simulink model "Assignment_2_1_simulink"  (R2025a)
settings: Solver=FixedStepDiscrete  StartTime=0.0  StopTime=inf  FixedStep=0.1  RelTol=1e-3  EnableMultiTasking=on
model workspace (MAT data in the model file):
  Logfile_Data_Object : ros2bag (value not decoded)
  Logfile_Path = '/home/diego/Desktop/Assignments/GitHub/ASSIGNMENT_2/tb3_subset/metadata.yaml'
  Logfile_Playback_Duration = nan
  Logfile_Playback_Offset = nan
values from neighbouring files (symbols this model uses):
  Kv = 0.8    [Assignment_2.m]
  Kw = 2    [Assignment_2.m]
  Quaternion_Matrix = [waypoints(:, 1:2) Quaternion_Matrix]    [Assignment_2.m]
  tol = 0.05    [Assignment_2.m]
undefined symbols (not defined in the file or in its folder): twist
libraries: ros2lib x5
settings Model: Creator=arrigon88_msi_u24  LastModifiedBy=diego
settings OptimizationCC: DefaultParameterBehavior=Inlined  EnhancedBackFolding=on  PassReuseOutputArgsAs=Individual arguments  ZeroExternalMemoryAtStartup=off  ZeroInternalMemoryAtStartup=off  MaxStackSize=64  OptimizeBlockOrder=speed  DifferentSizesBufferReuse=on  OptimizationCustomize=off  EfficientTunableParamExpr=on
settings DebuggingCC: ParameterTunabilityLossMsg=error
settings HardwareCC: ProdBitPerLong=64.0  ProdHWDeviceType=Intel->x86-64 (Linux 64)
settings SFSimCC: MATLABDynamicMemAlloc=off
settings RTWCC: SystemTargetFile=ert.tlc  HardwareBoard=Robot Operating System 2 (ROS 2)  TLCOptions="-aInlineSetEventsForThisBaseRateFcn=TLC_FALSE -aSuppressMultiTaskScheduler=TLC_FALSE  -aRateBasedStepFcn=0"  TemplateMakefile=ert_default_tmf  Toolchain=Colcon Tools  TargetLang=C++  Description=Embedded Coder
settings CodeAppCC: ForceParamTrailComments=on  IgnoreCustomStorageClasses=off  OperatorAnnotations=on  SimulinkDataObjDesc=on  SFDataObjDesc=on  InsertBlockDesc=on
settings ERTTargetCC: ExtModeTransport=2.0  ExtModeAutomaticAllocSize=off  RootIOFormat=Structure reference  CodeInterfacePackaging=C++ class

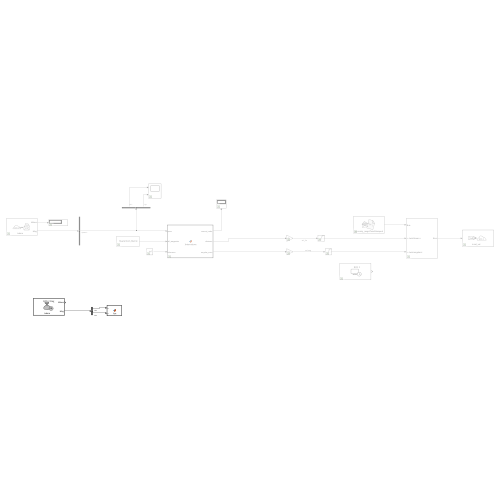
[thumbnail: Simulink's stored preview of the top-level diagram]
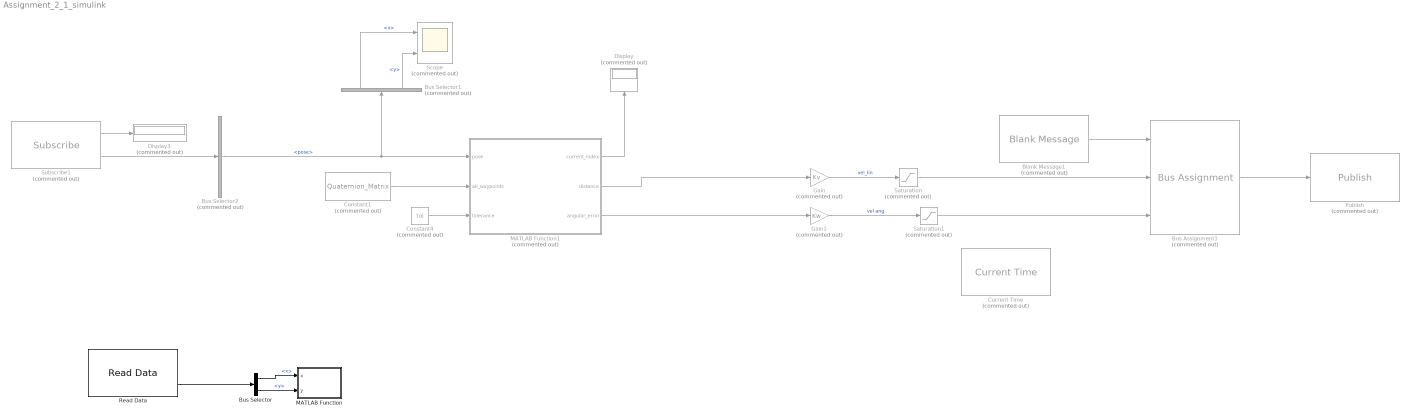
== system Assignment_2_1_simulink ==
  Blank Message1 : ros2lib/Blank Message  Commented=on  messageClass=Message  entityType=geometry_msgs/TwistStamped  messageType=geometry_msgs/TwistStamped  SampleTime=inf
  Bus Assignment1 : BusAssignment  Commented=on  AssignedSignals=twist.linear.x,twist.angular.z
  Bus Selector : BusSelector  OutputSignals=pose.pose.position.x,pose.pose.position.y
  Bus Selector1 : BusSelector  Commented=on  OutputSignals=pose.position.x,pose.position.y
  Bus Selector2 : BusSelector  Commented=on  OutputSignals=pose
  Constant1 : Constant  Commented=on  Value=Quaternion_Matrix
  Constant4 : Constant  Commented=on  Value=tol
  Current Time : ros2lib/Current Time  Commented=on  OutputFormat=double  SampleTime=-1  ModelName=Assignment_2_simulink
  Display : Display  Commented=on
  Display3 : Display  Commented=on
  Gain : Gain  Commented=on  Gain=Kv
  Gain1 : Gain  Commented=on  Gain=Kw
  MATLAB Function : MATLAB Function  TreatAsAtomicUnit=on
  MATLAB Function1 : MATLAB Function  Commented=on  TreatAsAtomicUnit=on
  Publish : ros2lib/Publish  Commented=on  topicSource=Select from ROS network  topic=/cmd_vel  messageType=geometry_msgs/TwistStamped  QOSHistory=Keep last  QOSDepth=10  QOSReliability=Reliable  QOSDurability=Volatile  QOSDeadline=Inf  QOSLifespan=Inf  QOSLiveliness=Automatic  QOSLeaseDuration=Inf  QOSAvoidROSNamespaceConventions=off
  Read Data : ros2lib/Read Data  topic=/odom  sampleTime=-1  logfileType=rosbag2  modelName=Assignment_2_1_simulink  msgType=nav_msgs/Odometry
  Saturation : Saturate  Commented=on  UpperLimit=0.2  LowerLimit=0
  Saturation1 : Saturate  Commented=on  UpperLimit=0.4  LowerLimit=0
  Scope : Scope  Commented=on  NumInputPorts=2
      settings: ActiveDisplayYMinimum=-7.8774180960192659  ActiveDisplayYMaximum=6.4713068809857548
  Subscribe1 : ros2lib/Subscribe  Commented=on  topicSource=Select from ROS network  topic=/odom  messageType=nav_msgs/Odometry  sampleTime=-1  QOSHistory=Keep last  QOSDepth=10  QOSReliability=Reliable  QOSDurability=Volatile  QOSDeadline=Inf  QOSLifespan=Inf  QOSLiveliness=Automatic  QOSLeaseDuration=Inf  QOSAvoidROSNamespaceConventions=off
  wires:
  MATLAB Function1/1(current_index) -> Display/1
  Subscribe1/2 -> Bus Selector2/1
  Subscribe1/1 -> Display3/1
  Constant4/1 -> MATLAB Function1/3(tolerance)
  MATLAB Function1/2(distance) -> Gain/1
  Gain/1 -> Saturation/1  "vel_lin"
  MATLAB Function1/3(angular_error) -> Gain1/1
  Gain1/1 -> Saturation1/1  "vel ang"
  Saturation/1 -> Bus Assignment1/2
  Blank Message1/1 -> Bus Assignment1/1
  Bus Assignment1/1 -> Publish/1
  Saturation1/1 -> Bus Assignment1/3
  Bus Selector2/1 -> Bus Selector1/1, MATLAB Function1/1(pose)  "<pose>"
  Bus Selector1/2 -> Scope/2  "<y>"
  Bus Selector1/1 -> Scope/1  "<x>"
  Constant1/1 -> MATLAB Function1/2(all_waypoints)
  Read Data/2 -> Bus Selector/1
  Bus Selector/1 -> MATLAB Function/1(x)  "<x>"
  Bus Selector/2 -> MATLAB Function/2(y)  "<y>"

== matlab function Assignment_2_1_simulink/MATLAB Function1 ==
  data: pose input; current_index output; all_waypoints input; tolerance input; distance output; angular_error output
function [current_index, distance, angular_error] = Interruttore(pose, all_waypoints, tolerance)
    
   % -----------------------------------------------------------------
    
    % Dichiara 'index' come persistente (mantiene il valore tra le chiamate)
    persistent index;
    
    % Inizializza 'index' solo alla prima chiamata (quando e' vuoto)
    if isempty(index)
        index = 1; % Inizia dal primo waypoint
    end

    % Ottieni il numero totale di waypoint per sicurezza
    num_waypoints = size(all_waypoints, 1);

    % Assicurati che l'indice non superi il massimo
    % (se siamo arrivati all'ultimo, rimaniamo li)
    if index > num_waypoints
        index = num_waypoints;
    end
    
    % -----------------------------------------------------------------
    % 2. ESECUZIONE LOGICA
    % -----------------------------------------------------------------
    
    % Estrai il target CORRENTE usando l'indice interno
    target = all_waypoints(index, :);
    
    % Assegna l'output: 'current_index' e' l'indice che stiamo processando
    current_index = index;

    % --- Preparazione ---
    pos_attuale = [pose.pose.position.x, pose.pose.position.y];
    pos_target = [target(1), target(2)];
    angular_error = 0; % Valore di default (risolve l'errore Coder)

    q_current = [pose.pose.orientation.x; 
                 pose.pose.orientation.y; 
                 pose.pose.orientation.z; 
                 pose.pose.orientation.w];
             
    q_target = target(3:6)'; 

    % --- Calcolo Distanza ---
    distance = norm(pos_attuale - pos_target);
    
    % --- Logica di Passaggio Waypoint ---
    if distance < tolerance
       distance = 0; 
       
       % ... (Calcolo del quaternione di errore, come prima) ...
       q_current_inv = [-q_current(1); -q_current(2); -q_current(3); q_current(4)];
       x1 = q_target(1); y1 = q_target(2); z1 = q_target(3); w1 = q_target(4);
       x2 = q_current_inv(1); y2 = q_current_inv(2); z2 = q_current_inv(3); w2 = q_current_inv(4);
       q_error = zeros(4, 1);
       q_error(4) = w1*w2 - x1*x2 - y1*y2 - z1*z2; % W
       q_error(1) = w1*x2 + x1*w2 + y1*z2 - z1*y2; % X
       q_error(2) = w1*y2 - x1*z2 + y1*w2 + z1*x2; % Y
       q_error(3) = w1*z2 + x1*y2 - y1*x2 + z1*w2; % Z
       
       angular_error = norm(q_error(1:3)); 
       
       % Se l'orientamento e' corretto...
       if angular_error < deg2rad(0.0001)
          % ...passa al prossimo waypoint (per il prossimo ciclo)
          if index < num_waypoints
             index = index + 1; 
          end
          angular_error = 0; 
       end
    end
    
    % Se non entriamo nell'IF, 'angular_error' rimane 0 (corretto per Kp)
    % e 'index' rimane invariato per il prossimo ciclo.
end

== matlab function Assignment_2_1_simulink/MATLAB Function ==
  data: x input; y input
function fcn(x , y)

plot(x,y);
